simulink model "Hopper_Land_Sim"  (R2023b)
settings: Solver=VariableStepAuto  StartTime=0.0  StopTime=64.5  FixedStep=0.1  MaxStep=0.1  RelTol=1e-6  AbsTol=1e-8
values from neighbouring files (symbols this model uses):
  c_l = 2*sqrt(k_l*m_leg)    [SpringModels.m]
  c_s = 2    [SpringModels.m]
  c_T = 90000    [SpringModels.m]
  C_T = 0.1    [Vehicle_Properties.m]
  g = 1.625    [CalculateLQRGains.m]    (also in IterativeLQR.m; LQR_Controller.m; Trap2D.m = param.g; Vehicle_Properties.m)
  k_l = 100000000000    [SpringModels.m]
  k_s = 500    [SpringModels.m]
  k_T = 9999999    [SpringModels.m]    (also in Vehicle_Properties.m = 0.8)
  K_x = K    [LQR_Controller.m]
  K_y = [K(1), -K(2), K(3), -K(4)]    [LQR_Controller.m]
  l = 4.2926/2    (= 2.1463)    [CalculateLQRGains.m]    (also in IterativeLQR.m; LQR_Controller.m; Vehicle_Properties.m)
  m_e = 150    [CalculateLQRGains.m]    (also in IterativeLQR.m; LQR_Controller.m; Vehicle_Properties.m)
  m_l = 803    [CalculateLQRGains.m]    (also in IterativeLQR.m; LQR_Controller.m; Vehicle_Properties.m)
  m_leg = 10    [SpringModels.m]
  m_s = 355.9/2    (= 177.95)    [SpringModels.m]
  mu_floor = .2    (= 0.2)    [SpringModels.m]
  mu_surface = 0.2    [Vehicle_Properties.m]
  n_floor = [cosd(90+floor_angle), 0, sind(90+floor_angle)]    [FloorModel.m]
  n_surface = [0; 0; 1]    [Vehicle_Properties.m]
  p_l2 = [1; 0; -.5]    [SpringModels.m]
  p_l3 = [0; -1; -.5]    [SpringModels.m]
  p_l4 = [0; 1; -.5]    [SpringModels.m]
  r_l1 = [cosd(angle_legs); 0; sind(leg_length)]    [FloorModel.m]    (also in SpringModels.m = r_l1/norm(r_l1))
  r_l2 = [-cosd(angle_legs); 0; sind(leg_length)]    [FloorModel.m]    (also in SpringModels.m = r_l2/norm(r_l2))
  r_l3 = [0; cosd(angle_legs); sind(leg_length)]    [FloorModel.m]    (also in SpringModels.m = r_l3/norm(r_l3))
  r_l4 = [0; -cosd(angle_legs); sind(leg_length)]    [FloorModel.m]    (also in SpringModels.m = r_l4/norm(r_l4))
libraries: matrix_library x17, slpidlib x5, simulink x2, simulink_extras x1, shared6dof x1, vrlib x1
(part 2 of 2)

== matlab function Hopper_Land_Sim/Controller/X-Y control/junk/MATLAB Function ==
  settings: updateMethod=DISCRETE
  data: Tx output; state input; last_control input; next_control output
function [Tx,next_control]  = getAction(state,last_control)
% Param defintion
n_samples = 200000;    % Number of rollout trajectories
horizon = 5;       % Prediction horizon represented as number of steps
lambda = 100;        % Temperature - Selectiveness of trajectories by their costs (The closer this value to 0, the "more" we take in considiration controls with less cost), 0 mean use control with best cost, huge value will lead to just taking mean of all trajectories without cost consideration
nu = 100;           % Exploration variance
R_v = .01;   % Control weighting matrix
cov_d = 500;     % Variance of control inputs disturbance 
dt = 0.05;           % Time step of controller and simulation
max_force = 2500;
goal_state = [0, 0, 0, 0];

control_sequence = last_control;

init_state = state;
S = zeros(n_samples, 1);

rollouts_states = zeros(n_samples, horizon+1, 4);
rollouts_costs = zeros(n_samples,1);

delta_u_1 = normrnd(0, cov_d, [n_samples, horizon]);

delta_u = zeros(1,n_samples,horizon);
delta_u(1,:,:) = delta_u_1;

for k = 1:n_samples
    prediction_state = zeros(4, horizon+1);
    prediction_state(:,1) = init_state;
    for i = 1:horizon                  
        % Single trajectory step
        prediction_state(:,i+1) = Step(control_sequence(i) + delta_u(1, k, i), dt, prediction_state(:,i));
                    
        % Compute cost of the state
        S(k) = S(k) + cost_function(prediction_state(:,i+1), control_sequence(i), delta_u(1, k, i), goal_state,nu,R_v);
    end
    rollouts_states(k,:,:) = prediction_state';
    rollouts_costs(k) = S(k);
end
S_normalized = S - min(S);

for i = 1:horizon
    control_sequence(i) = control_sequence(i) + total_entropy(lambda, delta_u(:,:,i)', S_normalized(:))'; 
end

% Add control saturation

control_sequence(control_sequence(:) > max_force) = max_force;
control_sequence(control_sequence(:) < -max_force) = -max_force;

action = control_sequence(1);

Tx = action(1);

next_control = [control_sequence(2:end) 0];

    function cost = cost_function(state, u, du, goal_state,nu,R_v)
        weight_states = diag([0,10000,0,2000000]);
        state_cost = (goal_state - state')*weight_states*(goal_state - state')';
        control_cost =  (1-1/nu)/2 * du'*R_v*du;
                % control_cost =  0;

        cost = state_cost + control_cost;
    end
    function value = total_entropy(lambda, du, trajectory_cost)
        exponents = exp(-1/lambda * trajectory_cost);
        value = sum(exponents.*du ./ sum(exponents),1);
    end
function next_state = Step(action, dt, state)
    m_l = 803; %kg
    m_e = 150;
    g = 1.625;
    l = 4.2926/2;

    x = state(1);
    phi = state(2);
    x_dot = state(3);
    phi_dot = state(4);
    T = action;

    x_ddot = (m_l*g*sin(phi)*cos(phi) - m_l*l*phi_dot^2*sin(phi)) / (m_e+m_l*(sin(phi)^2));
    phi_ddot = x_ddot*cos(phi)/l + g/l*sin(phi);

A_nonl = [x_dot;
         phi_dot;
         x_ddot;
         phi_ddot];
B_nonl = [0;
          0;
          T/(m_e+m_l*(sin(phi)^2));
          T*cos(phi)/(l*(m_e+m_l*(sin(phi)^2)))];

X_dot = A_nonl + B_nonl;
next_state = X_dot*dt + state;

end
        
end

== matlab function Hopper_Land_Sim/Controller/X-Y control/MATLAB Function1 ==
  settings: updateMethod=DISCRETE
  data: Tx output; state input; last_control input; next_control output
function [Tx,next_control]  = getAction(state,last_control)
% Param defintion
n_samples = 20000;    % Number of rollout trajectories
horizon = 25;       % Prediction horizon represented as number of steps
lambda = 15;        % Temperature - Selectiveness of trajectories by their costs (The closer this value to 0, the "more" we take in considiration controls with less cost), 0 mean use control with best cost, huge value will lead to just taking mean of all trajectories without cost consideration
nu = 1;           % Exploration variance
R_v = .01;   % Control weighting matrix
cov_d = 50;     % Variance of control inputs disturbance 
dt = 0.1;           % Time step of controller and simulation
max_force = 700;
goal_state = [0, 0, 0, 0];


Tx_initial = last_control(1);

control_sequence = repmat(Tx_initial,1,horizon);

init_state = state;
S = zeros(n_samples, 1);

rollouts_states = zeros(n_samples, horizon+1, 4);
rollouts_costs = zeros(n_samples,1);

delta_u_1 = normrnd(0, cov_d, [n_samples, horizon]);

delta_u = zeros(1,n_samples,horizon);
delta_u(1,:,:) = delta_u_1;

for k = 1:n_samples
    prediction_state = zeros(4, horizon+1);
    prediction_state(:,1) = init_state;
    for i = 1:horizon                  
        % Single trajectory step
        prediction_state(:,i+1) = Step(control_sequence(:,i) + delta_u(:, k, i), dt, prediction_state(:,i));
                    
        % Compute cost of the state
        S(k) = S(k) + cost_function(prediction_state(:,i+1), control_sequence(:,i), delta_u(:, k, i), goal_state,nu,R_v);
    end
    rollouts_states(k,:,:) = prediction_state';
    rollouts_costs(k) = S(k);
end
S_normalized = S - min(S);

for i = 1:horizon
    control_sequence(:,i) = control_sequence(:,i) + total_entropy(lambda, delta_u(:,:,i)', S_normalized(:))'; 
end

% Add control saturation

control_sequence(1, control_sequence(1,:) > max_force) = max_force;
control_sequence(1, control_sequence(1,:) < -max_force) = -max_force;

action = control_sequence(:,1);

Tx = action(1);

next_control = action;

    function cost = cost_function(state, u, du, goal_state,nu,R_v)
        weight_states = diag([0, 1000, 0, 100]);
        state_cost = (goal_state - state')*weight_states*(goal_state - state')';
        control_cost =  (1-1/nu)/2 * du'*R_v*du;
        cost = state_cost + control_cost;
    end
    function value = total_entropy(lambda, du, trajectory_cost)
        exponents = exp(-1/lambda * trajectory_cost);
        value = sum(exponents.*du ./ sum(exponents),1);
    end
function next_state = Step(action, dt, state)
    m_l = 803; %kg
    m_e = 150;
    g = 1.625;
    l = 4.2926/2;

    x = state(1);
    phi = state(2);
    x_dot = state(3);
    phi_dot = state(4);
    T = action;

    x_ddot = (m_l*g*sin(phi)*cos(phi) - m_l*l*phi_dot^2*sin(phi)) / (m_e+m_l*(sin(phi)^2));
    phi_ddot = x_ddot*cos(phi)/l + g/l*sin(phi);

A_nonl = [x_dot;
     phi_dot;
     x_ddot;
     phi_ddot];
B_nonl = [0;
          0;
          T/(m_e+m_l*(sin(phi)^2));
          T*cos(phi)/(l*(m_e+m_l*(sin(phi)^2)))];

X_dot = A_nonl + B_nonl;
next_state = X_dot*dt + state;

end
        
end
